simulink model "SOX_estimators"  (R2024a)
settings: Solver=FixedStepAuto  StartTime=0.0  StopTime=inf  RelTol=1e-3
values from neighbouring files (symbols this model uses):
  SOH_ESTIM_INIT = 1.0    [SOXDictionary.sldd]    (also in SOXDictionaryGotion.sldd = 1.0
  TOTAL_N_CELL_VOLTAGE = 24    [SOXDictionary.sldd]
settings Model: DataDictionary=SOXDictionary.sldd  SimulationMode=accelerator  Creator=mmackenzie  LastModifiedBy=mmackenzie

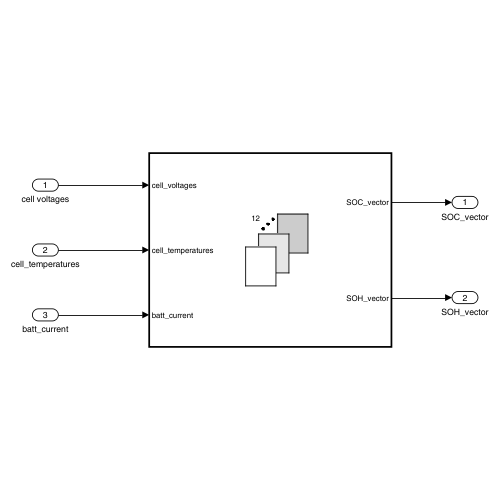
[thumbnail: Simulink's stored preview of the top-level diagram]
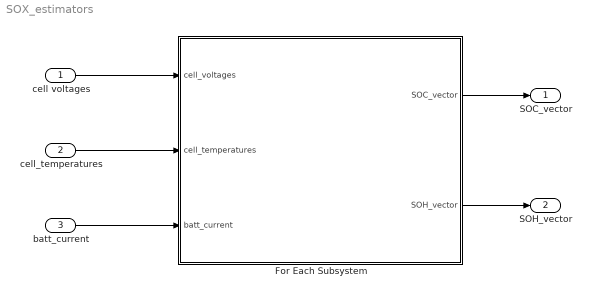
== system SOX_estimators ==
  cell voltages : Inport  OutDataTypeStr=uint16  PortDimensions=[TOTAL_N_CELL_VOLTAGE,1]
  cell_temperatures : Inport  Port=2  OutDataTypeStr=int16  PortDimensions=[TOTAL_N_CELL_VOLTAGE,1]
  batt_current : Inport  Port=3  OutDataTypeStr=int32  PortDimensions=1
  For Each Subsystem : Subsystem  TreatAsAtomicUnit=on
  SOC_vector : Outport  OutDataTypeStr=uint16  PortDimensions=[TOTAL_N_CELL_VOLTAGE,1]
  SOH_vector : Outport  Port=2  OutDataTypeStr=uint16  PortDimensions=[TOTAL_N_CELL_VOLTAGE,1]
  wires:
  cell voltages/1 -> For Each Subsystem/1(cell_voltages)
  cell_temperatures/1 -> For Each Subsystem/2(cell_temperatures)
  batt_current/1 -> For Each Subsystem/3(batt_current)
  For Each Subsystem/2(SOH_vector) -> SOH_vector/1
  For Each Subsystem/1(SOC_vector) -> SOC_vector/1

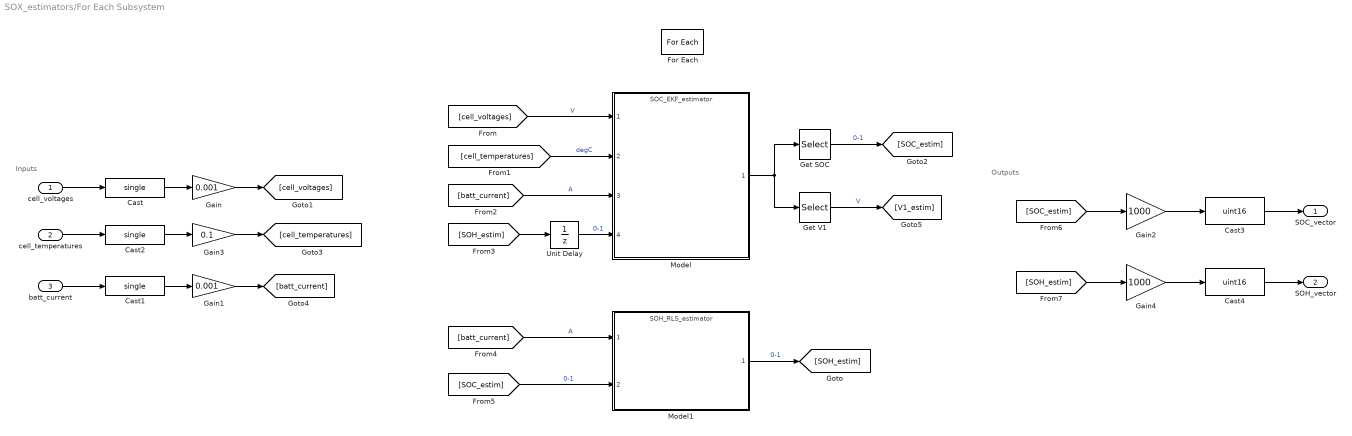
== system SOX_estimators/For Each Subsystem ==
  note: Outputs
  note: Inputs
  cell_voltages : Inport  OutDataTypeStr=uint16  PortDimensions=1  Partition=on  PartitionDimension=1  PartitionWidth=1  PartitionOffset=0
  cell_temperatures : Inport  Port=2  OutDataTypeStr=int16  PortDimensions=1  Partition=on  PartitionDimension=1  PartitionWidth=1  PartitionOffset=0
  batt_current : Inport  Port=3  OutDataTypeStr=int32  PortDimensions=1
  Cast : DataTypeConversion  OutDataTypeStr=single  SaturateOnIntegerOverflow=off  RndMeth=Floor
  Cast1 : DataTypeConversion  OutDataTypeStr=single  SaturateOnIntegerOverflow=off  RndMeth=Floor
  Cast2 : DataTypeConversion  OutDataTypeStr=single  SaturateOnIntegerOverflow=off  RndMeth=Floor
  Cast3 : DataTypeConversion  OutDataTypeStr=uint16  SaturateOnIntegerOverflow=off  RndMeth=Floor
  Cast4 : DataTypeConversion  OutDataTypeStr=uint16  SaturateOnIntegerOverflow=off  RndMeth=Floor
  For Each : ForEach  DisableCoverage=on
  Gain : Gain  Gain=0.001
  Gain1 : Gain  Gain=0.001
  Gain2 : Gain  Gain=1000
  Gain3 : Gain  Gain=0.1
  Gain4 : Gain  Gain=1000
  Get SOC : Selector  InputPortWidth=4  IndexOptions=Index vector (dialog)  Indices=1  OutputSizes=1
  Get V1 : Selector  InputPortWidth=4  IndexOptions=Index vector (dialog)  Indices=2  OutputSizes=1
  Model : ModelReference  ModelNameDialog=SOC_EKF_estimator.slx  SimulationMode=Normal  ModelReferenceVersion=1.53
  Model1 : ModelReference  ModelNameDialog=SOH_RLS_estimator.slx  SimulationMode=Normal  ModelReferenceVersion=1.51
  Unit Delay : UnitDelay  InitialCondition=SOH_ESTIM_INIT  SampleTime=-1  HasFrameUpgradeWarning=on
  SOC_vector : Outport  OutDataTypeStr=uint16  PortDimensions=1  ConcatenationDimension=1
  SOH_vector : Outport  Port=2  OutDataTypeStr=uint16  PortDimensions=1  ConcatenationDimension=1
  wires:
  [SOC_estim] -> Gain2/1
  [cell_voltages] -> Model/1  "V"
  Model1/1 -> [SOH_estim]  "0-1"
  Cast/1 -> Gain/1
  Gain1/1 -> [batt_current]
  Gain/1 -> [cell_voltages]
  cell_temperatures/1 -> Cast2/1
  batt_current/1 -> Cast1/1
  Gain3/1 -> [cell_temperatures]
  Cast1/1 -> Gain1/1
  Cast2/1 -> Gain3/1
  cell_voltages/1 -> Cast/1
  [cell_temperatures] -> Model/2  "degC"
  [batt_current] -> Model/3  "A"
  [SOH_estim] -> Unit Delay/1
  Unit Delay/1 -> Model/4  "0-1"
  [batt_current] -> Model1/1  "A"
  Model/1 -> Get V1/1, Get SOC/1
  Get SOC/1 -> [SOC_estim]  "0-1"
  Get V1/1 -> [V1_estim]  "V"
  [SOC_estim] -> Model1/2  "0-1"
  [SOH_estim] -> Gain4/1
  Gain2/1 -> Cast3/1
  Gain4/1 -> Cast4/1
  Cast3/1 -> SOC_vector/1
  Cast4/1 -> SOH_vector/1
